simulink model "robot_capteur_etu"  (R2017a)
settings: Solver=VariableStepAuto  StartTime=0.0  StopTime=10.0  RelTol=1e-3
values from neighbouring files (symbols this model uses):
  K = -place(A,B,poles)    [matrices.m]    (also in simulation_robot.m = -place(A,B,V); simulation_robot_echant.m = -place(A,B,V))
  ue = 0    [simulation_robot.m]    (also in simulation_robot_echant.m)
  x0 = [0 pi/10 0 0]    [simulation_robot.m]    (also in simulation_robot_echant.m)
  xe = [0 0 0 0]    [simulation_robot.m]    (also in simulation_robot_echant.m)
settings Model: Creator=jky  LastModifiedBy=jky

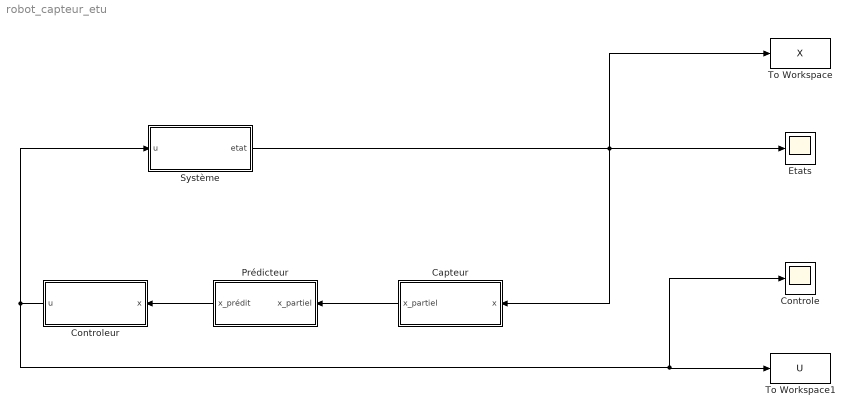
== system robot_capteur_etu ==
  Capteur : Subsystem
  Controle : Scope
  Controleur : Subsystem
  Etats : Scope
  Prédicteur : Subsystem
  Système : Subsystem
  To Workspace : ToWorkspace  VariableName=X  SaveFormat=Timeseries  SampleTime=-1
  To Workspace1 : ToWorkspace  VariableName=U  SaveFormat=Timeseries  SampleTime=-1
  wires:
  Système/1(etat) -> Capteur/1(x), To Workspace/1, Etats/1
  Controleur/1(u) -> Controle/1, To Workspace1/1, Système/1(u)
  Prédicteur/1("x_prédit ") -> Controleur/1(x)
  Capteur/1(x_partiel) -> Prédicteur/1(x_partiel)

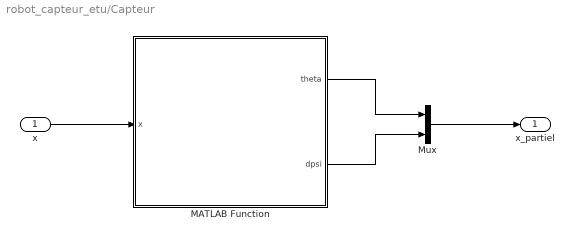
== system robot_capteur_etu/Capteur ==
  x : Inport
  MATLAB Function : MATLAB Function  TreatAsAtomicUnit=on
  Mux : Mux  Inputs=2
  x_partiel : Outport
  wires:
  x/1 -> MATLAB Function/1(x)
  MATLAB Function/1(theta) -> Mux/1
  MATLAB Function/2(dpsi) -> Mux/2
  Mux/1 -> x_partiel/1

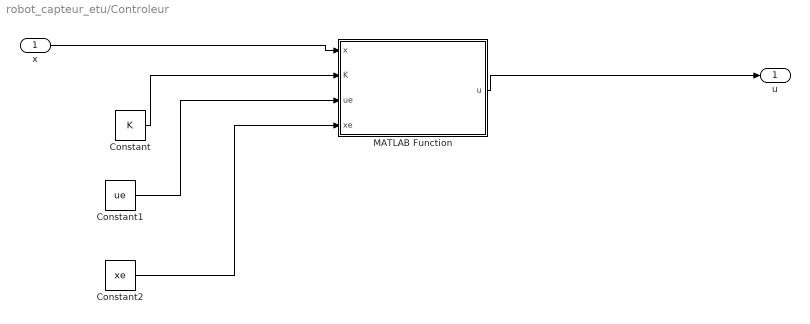
== system robot_capteur_etu/Controleur ==
  x : Inport
  Constant : Constant  Value=K
  Constant1 : Constant  Value=ue
  Constant2 : Constant  Value=xe
  MATLAB Function : MATLAB Function  TreatAsAtomicUnit=on
  u : Outport
  wires:
  x/1 -> MATLAB Function/1(x)
  MATLAB Function/1(u) -> u/1
  Constant/1 -> MATLAB Function/2(K)
  Constant1/1 -> MATLAB Function/3(ue)
  Constant2/1 -> MATLAB Function/4(xe)

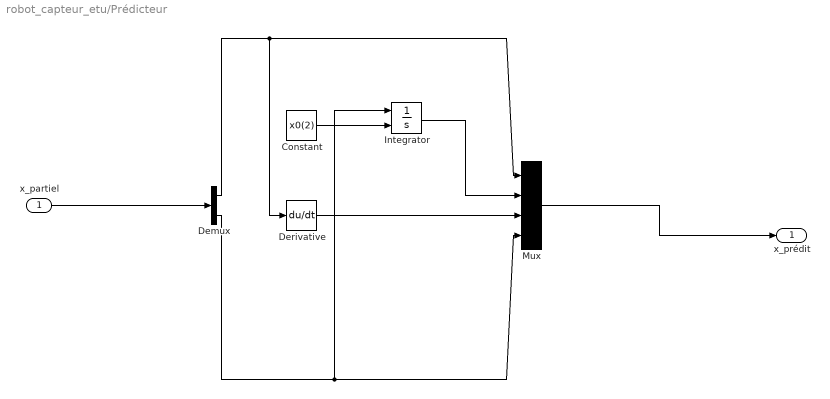
== system robot_capteur_etu/Prédicteur ==
  x_partiel : Inport
  Constant : Constant  Value=x0(2)
  Demux : Demux  Outputs=2
  Derivative : Derivative
  Integrator : Integrator  InitialConditionSource=external
  Mux : Mux
  "x_prédit " : Outport
  wires:
  Mux/1 -> "x_prédit "/1
  x_partiel/1 -> Demux/1
  Demux/1 -> Derivative/1, Mux/1
  Demux/2 -> Integrator/1, Mux/4
  Derivative/1 -> Mux/3
  Integrator/1 -> Mux/2
  Constant/1 -> Integrator/2

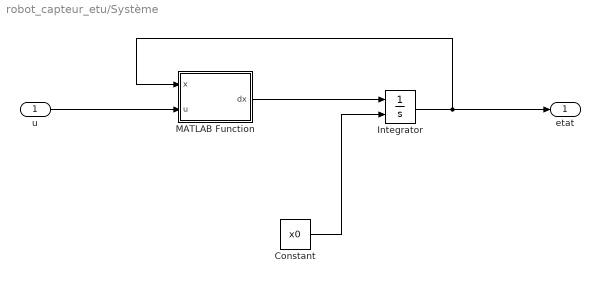
== system robot_capteur_etu/Système ==
  u : Inport
  Constant : Constant  Value=x0
  Integrator : Integrator  InitialConditionSource=external  InitialCondition=[pi/20 0]
  MATLAB Function : MATLAB Function  TreatAsAtomicUnit=on
  etat : Outport
  wires:
  u/1 -> MATLAB Function/2(u)
  Integrator/1 -> etat/1, MATLAB Function/1(x)
  MATLAB Function/1(dx) -> Integrator/1
  Constant/1 -> Integrator/2

== matlab function robot_capteur_etu/Controleur/MATLAB Function ==
  data: x input; u output; K input; ue input; xe input
function u = fcn(x, K, ue, xe)
u = ue + transpose(K)*(x-xe);

== matlab function robot_capteur_etu/Système/MATLAB Function ==
  data: x input; u input; dx output
function dx   = fonction( x, u)
%   Dynamic equations of motion of the segway on an axis.
%   Inputs: - x = [theta psi dtheta dpsi]
%               theta: average angle of the wheels      [rad]
%               psi: body pitch angle                   [rad]
%               dtheta: average velocity of the wheels  [rad/s]
%               dpsi: body pitch velocity               [rad/s]
%          - u: DC motor voltage (same value for both motors) [V]

    % State
    psi = x(2);
    dtheta = x(3);
    dpsi = x(4);

    % Parameters
    
    g = 9.81;           % gravity acceleration [m/sec^2]
    m = 0.03;           % wheel weight [kg]
    R = 0.04;           % wheel radius [m]
    Jw = m*R^2/2;       % wheel inertia moment [kg*m^2]
    M = 0.6;            % body weight [kg]
    H = 0.144;          % body height [m]
    L = H/2;            % distance of the center of mass from the wheel axle [m]
    Jpsi = M*L^2/3;     % body pitch inertia [kgm^2]
    Jm = 1e-5;          % DC motor inertia moment [kgm^2]
    Rm = 6.69;          % DC motor resistance [Ohm]
    Kb = 0.468;         % DC motor back EMF constant [Vsec/rad]
    Kt = 0.317;         % DC motor torque constant [Nm/A]
    n = 1;              % gear ratio
    fm = 0.0022;        % friction coefficient between body and DC motor
    fw = 0;             % friction coefficient between wheel and floor
    
    % Equations of motion
    c1 = (2*m+M)*R^2 + 2*Jw + 2*n^2*Jm;
    c2 = M*L*R*cos(psi) - 2*n^2*Jm;
    c3 = -M*L*R*dpsi^2*sin(psi);
    c4 = M*L^2 + Jpsi + 2*n^2*Jm;
    c5 = -M*g*L*sin(psi);

    alpha = Kt/Rm;
    beta = Kt*Kb/Rm + fm;

    Ftheta = alpha*(2*u) - 2*(beta+fw)*dtheta + 2*beta*dpsi;
    Fpsi = -alpha*(2*u) + 2*beta*dtheta - 2*beta*dpsi;

    ddtheta = (c4*c3 - c2*c5 + c4*Ftheta - c2*Fpsi)/(c4*c1 - c2^2);
    ddpsi = (Fpsi- c2*ddtheta - c5)/c4;
    dx = [dtheta dpsi ddtheta ddpsi]';

end

== matlab function robot_capteur_etu/Capteur/MATLAB Function ==
  data: x input; theta output; dpsi output
function [theta,dpsi] = fcn(x)

theta = x(1);
dpsi = x(4);
